simulink model "cpg_optimized"  (R2016a)
settings: Solver=FixedStepAuto  StartTime=0.0  StopTime=inf  FixedStep=0.04  RelTol=1e-3
values from neighbouring files (symbols this model uses):
  A_f = 0.1    [setup.m]
  ICNotPresent = 1    [setup.m]
  joints_in_use = [j_i_m('l_leg_hpx') j_i_m('l_leg_hpy') j_i_m('l_leg_kny') j_i_m('l_leg_aky') j_i_m('l_leg_akx') j_i_m('l_arm_shx') j_i_m('r_leg_hpx') j_i_m('r_leg_hpy') j_i_m('r_leg_kny') j_i_m('r_leg_aky') j_i_m('r_leg_akx') j_i_m('r_arm_shx')]    [setup.m]
  sigma_f = 2.2    [setup.m]
  sigma_s = 1    [setup.m]
  t_m = 0.1    [setup.m]
  t_s = 2    [setup.m]
undefined symbols (not defined in the file or in its folder): DiscIntNeverNeededParam, get, Position, SendJointCommand, SetThisJoint
libraries: fuzblock x72, dspsnks4 x4, simulink x2, robotlib x2, dspsrcs4 x1, dspindex x1, sldrtlib x1
(part 1 of 2)
settings Model: SimulationMode=accelerator  Creator=batyr  LastModifiedBy=batyr
settings SolverCC: EnableConcurrentExecution=on
settings DataIOCC: FinalStateName=CPGSimFinalState  LimitDataPoints=on  SaveCompleteFinalSimState=on  ReturnWorkspaceOutputs=on
settings OptimizationCC: BlockReduction=off  OptimizeBlockIOStorage=off  BufferReuse=off  GlobalBufferReuse=off  ExpressionFolding=off  LocalBlockOutputs=off  EfficientMapNaN2IntZero=off  OptimizeModelRefInitCode=on  MaxStackSize=64
settings DebuggingCC: ReadBeforeWriteMsg=DisableAll  WriteAfterWriteMsg=DisableAll  WriteAfterReadMsg=DisableAll  MultiTaskDSMMsg=none  AllowSymbolicDim=off
settings HardwareCC: ProdBitPerLong=64  ProdLargestAtomicFloat=None  ProdHWDeviceType=Intel->x86-64  TargetBitPerPointer=64  TargetLongLongMode=on  TargetIntDivRoundTo=Zero  TargetEndianess=LittleEndian  TargetWordSize=64  TargetHWDeviceType=MATLAB Host  ProdEqTarget=off
settings ModelReferenceCC: UpdateModelReferenceTargets=IfOutOfDate  PropagateSignalLabelsOutOfModel=off
settings SFSimCC: SFSimEcho=off
settings RTWCC: TargetLang=C++
settings CodeAppCC: MaxIdLength=128
settings GRTTargetCC: GeneratePreprocessorConditionals=Use local settings  CombineOutputUpdateFcns=off  GRTInterface=on

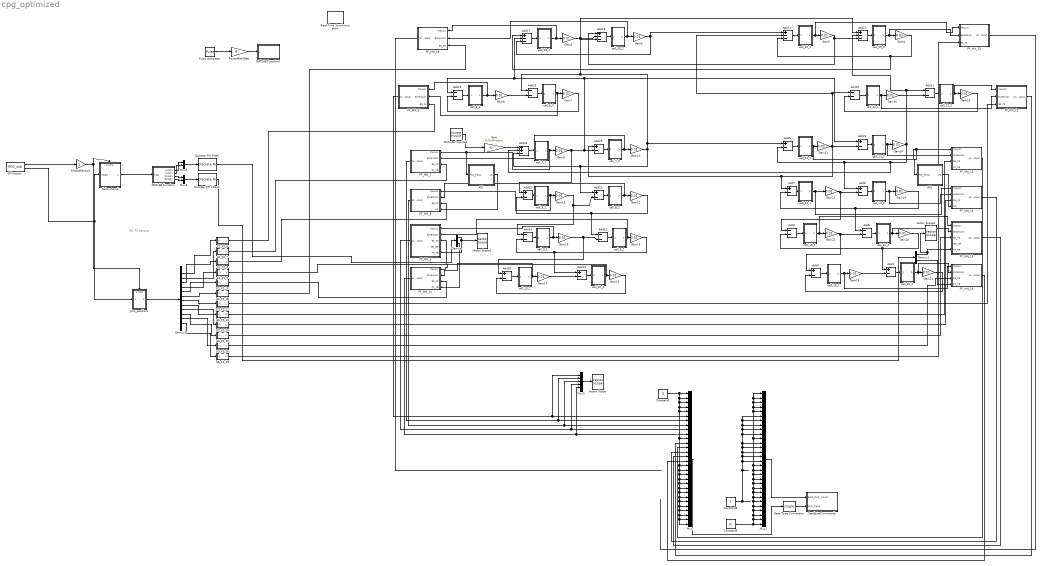
== system cpg_optimized ==
  note: ES, FS sensors
  AS1 : Subsystem
  AS2 : Subsystem
  Add{3,6,10..11,14..16,21} (8 alike) : Sum  Inputs=--
  Add{12..13,17..18} (4 alike) : Sum  Inputs=+--
  Add{4..5,7..9,19..20,22..23,25..26} (11 alike) : Sum  Inputs=+-
  Add24 : Sum  Inputs=++-
  Constant1 : Constant  Value=0  OutDataTypeStr=double
  Constant5 : Constant  Value=0  OutDataTypeStr=boolean
  Constant6 : Constant  OutDataTypeStr=boolean
  Data Type Conversion : DataTypeConversion  OutDataTypeStr=single
  Demux : Demux  Outputs=2
  Demux1 : Demux  Outputs=2
  Demux2 : Demux  Outputs=12
  Discrete Impulse2 : dspsrcs4/Discrete  Impulse  Delay=1  SampleTime=-1  FrameSample=1  OutputFrames=off  dataType=double  isSigned=on  wordLen=16  udDataType=sfix(16)  fracBitsMode=Best precision  numFracBits=15  OutDataTypeStr=double  LastOutDataTypeStr=double
  Discrete FIR Filter : DiscreteFir
  Discrete FIR Filter1 : DiscreteFir
  ES_FS_10 : Subsystem
  ES_FS_12 : Subsystem
  ES_FS_13 : Subsystem
  ES_FS_14 : Subsystem
  ES_FS_15 : Subsystem
  ES_FS_16 : Subsystem
  ES_FS_18 : Subsystem
  ES_FS_25 : Subsystem
  ES_FS_6 : Subsystem
  ES_FS_7 : Subsystem
  ES_FS_8 : Subsystem
  ES_FS_9 : Subsystem
  EnableSensors : Gain
  Gain : Gain  Gain=ICNotPresent
  Gain{3..26} (24 alike) : Gain  Gain=0.01
  Joint_positions : Subsystem
  MATLAB Function : MATLAB Function  TreatAsAtomicUnit=on
  MATLAB Function1 : MATLAB Function  TreatAsAtomicUnit=on
  Mux : Mux  Inputs=30
  Mux2 : Mux  Inputs=30
  Mux3 : Mux  Inputs=2
  Mux4 : Mux  Inputs=2
  Mux5 : Mux  Inputs=5
  PF_MN_10 : Subsystem
  PF_MN_12 : Subsystem
  PF_MN_13 : Subsystem
  PF_MN_14 : Subsystem
  PF_MN_15 : Subsystem
  PF_MN_16 : Subsystem
  PF_MN_18 : Subsystem
  PF_MN_25 : Subsystem
  PF_MN_6 : Subsystem
  PF_MN_7 : Subsystem
  PF_MN_8 : Subsystem
  PF_MN_9 : Subsystem
  PauseAfterStep : Gain  Gain=0
  Pulse Generator : DiscretePulseGenerator  PhaseDelay=1  SampleTime=-1
  Real-Time Synchronization : sldrtlib/Real-Time Synchronization  SampleTime=-1  MaxMissedTicks=100000  ShowMissedTicks=off  YieldWhenWaiting=off
  S-Function : S-Function  FunctionName=ROS_sub  SFunctionDeploymentMode=off  EnableBusSupport=off
  SendJointCommands : Subsystem
  Subsystem4 : Subsystem
  Vector Scope : dspsnks4/Vector Scope  ScopeProperties=on  Domain=Time  HorizSpan=1  DisplayProperties=off  AxisGrid=on  Memory=off  FrameNumber=on  AxisLegend=off  AxisZoom=off  OpenScopeAtSimStart=on  OpenScopeImmediately=off  FigPos=get(0,'defaultfigureposition')  AxisProperties=off  XUnits=Hertz  XRange=[0...Fs/2]  InheritXIncr=on  XIncr=1  XLabel=Time  XLimit=Auto  XMin=0  XMax=1  XStart=0  YUnits=dB  YLabel=Amplitude  LineProperties=off  XAxisParamsVer=6.9
      settings: YMin=-10  YMax=10
  Vector Scope1 : dspsnks4/Vector Scope  ScopeProperties=on  Domain=Time  HorizSpan=1  DisplayProperties=off  AxisGrid=on  Memory=off  FrameNumber=on  AxisLegend=off  AxisZoom=off  OpenScopeAtSimStart=on  OpenScopeImmediately=off  FigPos=get(0,'defaultfigureposition')  AxisProperties=off  XUnits=Hertz  XRange=[0...Fs/2]  InheritXIncr=on  XIncr=1  XLabel=Time  XLimit=Auto  XMin=0  XMax=1  XStart=0  YUnits=dB  YLabel=Amplitude  LineProperties=off  XAxisParamsVer=6.9
      settings: YMin=-10  YMax=10
  Vector Scope2 : dspsnks4/Vector Scope  ScopeProperties=on  Domain=Time  HorizSpan=1  DisplayProperties=off  AxisGrid=on  Memory=off  FrameNumber=on  AxisLegend=off  AxisZoom=off  OpenScopeAtSimStart=on  OpenScopeImmediately=off  FigPos=get(0,'defaultfigureposition')  AxisProperties=off  XUnits=Hertz  XRange=[0...Fs/2]  InheritXIncr=on  XIncr=1  XLabel=Time  XLimit=Auto  XMin=0  XMax=1  XStart=0  YUnits=dB  YLabel=Amplitude  LineProperties=off  XAxisParamsVer=6.9
      settings: YMin=-10  YMax=10
  cell_10_1 : Subsystem
  cell_10_2 : Subsystem
  cell_12_1 : Subsystem
  cell_12_2 : Subsystem
  cell_13_1 : Subsystem
  cell_13_2 : Subsystem
  cell_14_1 : Subsystem
  cell_14_2 : Subsystem
  cell_15_1 : Subsystem
  cell_15_2 : Subsystem
  cell_16_1 : Subsystem
  cell_16_2 : Subsystem
  cell_18_1 : Subsystem
  cell_18_2 : Subsystem
  cell_25_1 : Subsystem
  cell_25_2 : Subsystem
  cell_6_1 : Subsystem
  cell_6_2 : Subsystem
  cell_7_1 : Subsystem
  cell_7_2 : Subsystem
  cell_8_1 : Subsystem
  cell_8_2 : Subsystem
  cell_9_1 : Subsystem
  cell_9_2 : Subsystem
  wires:
  Add3/1 -> cell_15_1/1(In1)
  cell_15_2/1(Out1) -> PF_MN_15/2(Extension), Gain20/1
  cell_15_1/1(Out1) -> PF_MN_15/1(Flexion), Gain22/1
  cell_16_1/1(Out1) -> PF_MN_16/1(Flexion), Gain18/1
  cell_16_2/1(Out1) -> PF_MN_16/2(Extension), Gain21/1
  Add4/1 -> cell_16_2/1(In1)
  Add5/1 -> cell_16_1/1(In1)
  Add6/1 -> cell_15_2/1(In1)
  Add7/1 -> cell_14_1/1(In1)
  cell_14_2/1(Out1) -> PF_MN_14/2(Extension), Gain19/1
  cell_14_1/1(Out1) -> PF_MN_14/1(Flexion), Gain23/1
  Add8/1 -> cell_14_2/1(In1)
  Add9/1 -> cell_13_1/1(In1)
  Add26/1 -> cell_13_2/1(In1)
  cell_7_1/1(Out1) -> AS1/1(Hip_flexor), PF_MN_7/1(Flexion), Gain9/1
  cell_7_2/1(Out1) -> PF_MN_7/2(Extension), Gain10/1
  cell_12_2/1(Out1) -> PF_MN_12/1(Flexion), Gain25/1
  cell_12_1/1(Out1) -> PF_MN_12/2(Extension), Gain26/1
  Add10/1 -> cell_12_1/1(In1)
  Add11/1 -> cell_12_2/1(In1)
  Add12/1 -> cell_25_1/1(In1)
  Add13/1 -> cell_25_2/1(In1)
  Add14/1 -> cell_9_1/1(In1)
  cell_9_2/1(Out1) -> Gain13/1, PF_MN_9/2(Extension)
  cell_9_1/1(Out1) -> PF_MN_9/1(Flexion), Gain16/1
  cell_10_1/1(Out1) -> PF_MN_10/2(Extension), Gain17/1
  cell_10_2/1(Out1) -> PF_MN_10/1(Flexion), Gain14/1
  Add19/1 -> cell_10_2/1(In1)
  Add20/1 -> cell_10_1/1(In1)
  Add21/1 -> cell_9_2/1(In1)
  Add22/1 -> cell_8_1/1(In1)
  cell_8_2/1(Out1) -> PF_MN_8/2(Extension), Gain12/1
  cell_8_1/1(Out1) -> PF_MN_8/1(Flexion), Gain15/1
  Add23/1 -> cell_8_2/1(In1)
  Add24/1 -> cell_7_1/1(In1)
  Add25/1 -> cell_7_2/1(In1)
  cell_13_1/1(Out1) -> AS2/1(Hip_flexor), PF_MN_13/1(Flexion), Gain11/1
  cell_13_2/1(Out1) -> PF_MN_13/2(Extension), Gain24/1
  cell_6_2/1(Out1) -> PF_MN_6/2(Extension), Gain7/1
  cell_6_1/1(Out1) -> PF_MN_6/1(Flexion), Gain8/1
  Add15/1 -> cell_6_1/1(In1)
  Add16/1 -> cell_6_2/1(In1)
  Add17/1 -> cell_18_1/1(In1)
  Discrete Impulse2/1 -> Gain/1
  Add18/1 -> cell_18_2/1(In1)
  cell_18_1/1(Out1) -> PF_MN_18/1(Flexion), Gain3/1
  cell_18_2/1(Out1) -> PF_MN_18/2(Extension), Gain6/1
  cell_25_1/1(Out1) -> PF_MN_25/1(Flexion), Gain5/1
  cell_25_2/1(Out1) -> PF_MN_25/2(Extension), Gain4/1
  Gain3/1 -> Add13/1, Add18/2
  Gain4/1 -> Add17/1, Add12/3
  Gain5/1 -> Add18/1, Add13/3
  Gain6/1 -> Add12/1, Add17/3
  Gain7/1 -> Add15/2
  Gain8/1 -> Add16/2
  Gain9/1 -> Add15/1, Add17/2, Add26/1, Add25/2, Add22/1
  Gain10/1 -> Add18/3, Add16/1, Add9/1, Add24/3, Add23/1
  Gain11/1 -> Add12/2, Add10/1, Add7/1, Add25/1, Add26/2
  Gain12/1 -> Add22/2, Add21/1
  Gain13/1 -> Add14/2, Add19/1
  Gain14/1 -> Add20/2
  Gain15/1 -> Add14/1, Add23/2
  Gain16/1 -> Add20/1, Add21/2
  Gain17/1 -> Add19/2
  Gain18/1 -> Add4/2
  Gain19/1 -> Add7/2, Add6/1
  Gain20/1 -> Add3/2, Add4/1
  Gain21/1 -> Add5/2
  Gain22/1 -> Add6/2, Add5/1
  Gain23/1 -> Add8/2, Add3/1
  Gain24/1 -> Add24/2, Add8/1, Add9/2, Add13/2, Add11/1
  Gain25/1 -> Add10/2
  Gain26/1 -> Add11/2
  S-Function/2 -> Subsystem4/1(MsgIn), Joint_positions/1(Msg)
  Mux/1 -> Data Type Conversion/1
  Joint_positions/1(Out2) -> Demux2/1
  Demux2/1 -> ES_FS_6/1(In)
  Demux2/2 -> ES_FS_7/1(In)
  Demux2/4 -> ES_FS_9/1(In)
  Demux2/5 -> ES_FS_10/1(In)
  Demux2/6 -> ES_FS_18/1(In)
  Demux2/7 -> ES_FS_12/1(In)
  Demux2/8 -> ES_FS_13/1(In)
  Demux2/9 -> ES_FS_14/1(In)
  Demux2/10 -> ES_FS_15/1(In)
  Demux2/11 -> ES_FS_16/1(In)
  Demux2/12 -> ES_FS_25/1(In)
  Demux2/3 -> ES_FS_8/1(In)
  ES_FS_6/1(Out) -> PF_MN_6/3(ES_FS)
  ES_FS_7/1(Out) -> PF_MN_7/3(ES_FS)
  ES_FS_8/1(Out) -> PF_MN_8/3(ES_FS)
  ES_FS_9/1(Out) -> PF_MN_9/3(ES_FS)
  ES_FS_10/1(Out) -> PF_MN_10/3(ES_FS)
  ES_FS_18/1(Out) -> PF_MN_18/3(ES_FS)
  ES_FS_12/1(Out) -> PF_MN_12/3(ES_FS)
  ES_FS_13/1(Out) -> PF_MN_13/3(ES_FS)
  ES_FS_14/1(Out) -> PF_MN_14/3(ES_FS)
  ES_FS_15/1(Out) -> PF_MN_15/3(ES_FS)
  ES_FS_16/1(Out) -> PF_MN_16/3(ES_FS)
  ES_FS_25/1(Out) -> PF_MN_25/3(ES_FS)
  Mux2/1 -> SendJointCommands/1(Send_Joint_Value?)
  AS2/1(AS) -> PF_MN_14/4(AS)
  PF_MN_25/1(Joint_Output) -> ?
  PF_MN_12/1(Joint_Output) -> Mux/12
  PF_MN_13/1(Joint_Output) -> Mux/13
  PF_MN_14/1(Joint_Output) -> Mux/14
  PF_MN_15/1(Joint_Output) -> Mux/15
  PF_MN_16/1(Joint_Output) -> Mux/16
  PF_MN_6/1(Joint_Output) -> Mux5/1, Mux/6
  PF_MN_7/1(Joint_Output) -> Mux5/2, Mux/7
  PF_MN_8/1(Joint_Output) -> Mux5/3, Mux/8
  PF_MN_9/1(Joint_Output) -> Mux5/4, Mux/9
  PF_MN_10/1(Joint_Output) -> Mux5/5, Mux/10
  PF_MN_18/1(Joint_Output) -> ?
  Data Type Conversion/1 -> SendJointCommands/2(Joint_Value)
  Constant6/1 -> Mux2/16, Mux2/15, Mux2/14, Mux2/13, Mux2/12, Mux2/10, Mux2/9, Mux2/8, Mux2/6, Mux2/7
  Mux5/1 -> Vector Scope/1
  AS1/1(AS) -> PF_MN_8/4(AS)
  Constant5/1 -> Mux2/25, Mux2/18, Mux2/1, Mux2/2, Mux2/3, Mux2/4, Mux2/5, Mux2/11, Mux2/17, Mux2/19, Mux2/20, Mux2/21, Mux2/22, Mux2/23, Mux2/24, Mux2/26, Mux2/27, Mux2/28, Mux2/29, Mux2/30
  S-Function/1 -> EnableSensors/1
  Gain/1 -> Add24/1
  EnableSensors/1 -> Joint_positions/Enable, Subsystem4/Enable
  Mux4/1 -> Discrete FIR Filter/1
  Mux3/1 -> Discrete FIR Filter1/1
  Demux1/2 -> PF_MN_16/4(FF_FB)
  Demux1/1 -> Vector Scope2/1, PF_MN_15/5(FF_FB)
  MATLAB Function/3(RFootX) -> Mux3/1
  MATLAB Function/4(RFootY) -> Mux3/2
  MATLAB Function/1(LFootX) -> Mux4/1
  MATLAB Function/2(LFootY) -> Mux4/2
  Demux/1 -> Vector Scope1/1, PF_MN_9/5(FF_FB)
  Demux/2 -> PF_MN_10/4(FF_FB)
  Constant1/1 -> Mux/3, Mux/5, Mux/11, Mux/17, Mux/18, Mux/19, Mux/20, Mux/21, Mux/22, Mux/23, Mux/25, Mux/26, Mux/27, Mux/30, Mux/29, Mux/28, Mux/24, Mux/4, Mux/2, Mux/1
  Pulse Generator/1 -> PauseAfterStep/1
  PauseAfterStep/1 -> MATLAB Function1/1(u)
  Subsystem4/1(MsgOut) -> MATLAB Function/1(msg)
  Discrete FIR Filter/1 -> Demux/1
  Discrete FIR Filter1/1 -> Demux1/1

== system cpg_optimized/AS1 ==
  Hip_flexor : Inport
  Constant1 : Constant  Value=0
  Constant2 : Constant  Value=0.1
  Detect Decrease : simulink/Logic and Bit Operations/Detect Decrease  vinit=1  InputProcessing=Inherited  OutDataTypeStr=boolean
  Display2 : Display
  Display4 : Display
  If : If  IfExpression=u1
  If Action Subsystem1 : Subsystem  TreatAsAtomicUnit=on
  If Action Subsystem3 : Subsystem  TreatAsAtomicUnit=on
  Merge1 : Merge
  AS : Outport
  wires:
  If/2 -> If Action Subsystem1/Action
  Constant1/1 -> If Action Subsystem1/1(In1)
  If Action Subsystem1/1(Out1) -> Merge1/2
  Merge1/1 -> Display2/1, AS/1
  Hip_flexor/1 -> Detect Decrease/1, Display4/1
  Detect Decrease/1 -> If/1
  Constant2/1 -> If Action Subsystem3/1(In1)
  If/1 -> If Action Subsystem3/Action
  If Action Subsystem3/1(Out1) -> Merge1/1

== system cpg_optimized/AS2 ==
  Hip_flexor : Inport
  Constant1 : Constant  Value=0
  Constant2 : Constant  Value=0.1
  Detect Decrease : simulink/Logic and Bit Operations/Detect Decrease  vinit=0.0  InputProcessing=Inherited  OutDataTypeStr=boolean
  Display2 : Display
  Display4 : Display
  If : If  IfExpression=u1
  If Action Subsystem1 : Subsystem  TreatAsAtomicUnit=on
  If Action Subsystem3 : Subsystem  TreatAsAtomicUnit=on
  Merge1 : Merge
  AS : Outport
  wires:
  If/2 -> If Action Subsystem1/Action
  Constant1/1 -> If Action Subsystem1/1(In1)
  If Action Subsystem1/1(Out1) -> Merge1/2
  Merge1/1 -> Display2/1, AS/1
  Hip_flexor/1 -> Detect Decrease/1, Display4/1
  Detect Decrease/1 -> If/1
  Constant2/1 -> If Action Subsystem3/1(In1)
  If/1 -> If Action Subsystem3/Action
  If Action Subsystem3/1(Out1) -> Merge1/1

== system cpg_optimized/ES_FS_10 ==
  In : Inport
  ES : fuzblock/Membership  Functions/Sigmoidal MF  a=6.9767  c=-0.075465
  FS : fuzblock/Membership  Functions/Sigmoidal MF  a=-6.9767  c=-0.075465
  Mux : Mux  Inputs=2
  Out : Outport
  wires:
  FS/1 -> Mux/2
  In/1 -> ES/1, FS/1
  ES/1 -> Mux/1
  Mux/1 -> Out/1

== system cpg_optimized/ES_FS_12 ==
  In : Inport
  ES : fuzblock/Membership  Functions/Sigmoidal MF  a=5.7692  c=-0.075739
  FS : fuzblock/Membership  Functions/Sigmoidal MF  a=-5.7692  c=-0.075739
  Mux : Mux  Inputs=2
  Out : Outport
  wires:
  FS/1 -> Mux/2
  In/1 -> ES/1, FS/1
  ES/1 -> Mux/1
  Mux/1 -> Out/1

== system cpg_optimized/ES_FS_13 ==
  In : Inport
  ES : fuzblock/Membership  Functions/Sigmoidal MF  a=2.765  c=-0.2
  FS : fuzblock/Membership  Functions/Sigmoidal MF  a=-2.765  c=-0.2
  Mux : Mux  Inputs=2
  Out : Outport
  wires:
  FS/1 -> Mux/2
  In/1 -> ES/1, FS/1
  ES/1 -> Mux/1
  Mux/1 -> Out/1

== system cpg_optimized/ES_FS_14 ==
  In : Inport
  ES : fuzblock/Membership  Functions/Sigmoidal MF  a=-2.5532  c=0.45
  FS : fuzblock/Membership  Functions/Sigmoidal MF  a=2.5532  c=0.45
  Mux : Mux  Inputs=2
  Out : Outport
  wires:
  FS/1 -> Mux/2
  In/1 -> ES/1, FS/1
  ES/1 -> Mux/1
  Mux/1 -> Out/1

== system cpg_optimized/ES_FS_15 ==
  In : Inport
  ES : fuzblock/Membership  Functions/Sigmoidal MF  a=4.3478  c=-0.1
  FS : fuzblock/Membership  Functions/Sigmoidal MF  a=-4.3478  c=-0.1
  Mux : Mux  Inputs=2
  Out : Outport
  wires:
  FS/1 -> Mux/2
  In/1 -> ES/1, FS/1
  ES/1 -> Mux/1
  Mux/1 -> Out/1

== system cpg_optimized/ES_FS_16 ==
  In : Inport
  ES : fuzblock/Membership  Functions/Sigmoidal MF  a=6.9767  c=0.076658
  FS : fuzblock/Membership  Functions/Sigmoidal MF  a=-6.9767  c=0.076658
  Mux : Mux  Inputs=2
  Out : Outport
  wires:
  FS/1 -> Mux/2
  In/1 -> ES/1, FS/1
  ES/1 -> Mux/1
  Mux/1 -> Out/1

== system cpg_optimized/ES_FS_18 ==
  In : Inport
  ES : fuzblock/Membership  Functions/Sigmoidal MF  a=1.9108  c=-1.3087
  FS : fuzblock/Membership  Functions/Sigmoidal MF  a=-1.9108  c=-1.3087
  Mux : Mux  Inputs=2
  Out : Outport
  wires:
  FS/1 -> Mux/2
  In/1 -> ES/1, FS/1
  ES/1 -> Mux/1
  Mux/1 -> Out/1

== system cpg_optimized/ES_FS_25 ==
  In : Inport
  ES : fuzblock/Membership  Functions/Sigmoidal MF  a=1.9108  c=1.3088
  FS : fuzblock/Membership  Functions/Sigmoidal MF  a=-1.9108  c=1.3088
  Mux : Mux  Inputs=2
  Out : Outport
  wires:
  FS/1 -> Mux/2
  In/1 -> ES/1, FS/1
  ES/1 -> Mux/1
  Mux/1 -> Out/1

== system cpg_optimized/ES_FS_6 ==
  In : Inport
  Display : Display
  ES : fuzblock/Membership  Functions/Sigmoidal MF  a=5.7692  c=0.075814
  FS : fuzblock/Membership  Functions/Sigmoidal MF  a=-5.7692  c=0.075814
  Mux : Mux  Inputs=2
  Out : Outport
  wires:
  FS/1 -> Mux/2
  In/1 -> ES/1, FS/1
  ES/1 -> Display/1, Mux/1
  Mux/1 -> Out/1

== system cpg_optimized/ES_FS_7 ==
  In : Inport
  ES : fuzblock/Membership  Functions/Sigmoidal MF  a=2.765  c=-0.2
  FS : fuzblock/Membership  Functions/Sigmoidal MF  a=-2.765  c=-0.2
  Mux : Mux  Inputs=2
  Out : Outport
  wires:
  FS/1 -> Mux/2
  In/1 -> ES/1, FS/1
  ES/1 -> Mux/1
  Mux/1 -> Out/1

== system cpg_optimized/ES_FS_8 ==
  In : Inport
  ES : fuzblock/Membership  Functions/Sigmoidal MF  a=-2.5532  c=0.45
  FS : fuzblock/Membership  Functions/Sigmoidal MF  a=2.5532  c=0.45
  Mux : Mux  Inputs=2
  Out : Outport
  wires:
  FS/1 -> Mux/2
  In/1 -> ES/1, FS/1
  ES/1 -> Mux/1
  Mux/1 -> Out/1

== system cpg_optimized/ES_FS_9 ==
  In : Inport
  ES : fuzblock/Membership  Functions/Sigmoidal MF  a=4.3478  c=-0.1
  FS : fuzblock/Membership  Functions/Sigmoidal MF  a=-4.3478  c=-0.1
  Mux : Mux  Inputs=2
  Out : Outport
  wires:
  FS/1 -> Mux/2
  In/1 -> ES/1, FS/1
  ES/1 -> Mux/1
  Mux/1 -> Out/1

== system cpg_optimized/Joint_positions ==
  Msg : Inport
  Enable : EnablePort
  Bus Selector : BusSelector  OutputSignals=Joints
  Constant7 : Constant  Value=joints_in_use
  Variable Selector2 : dspindex/Variable Selector  NumInputs=1  rowsOrCols=Rows  IdxMode=Variable  Elements=[1 3]  ZerOneIdxMode=One-based  errmode=Clip Index  FillMode=on  FillValues=0
  Vector Scope : dspsnks4/Vector Scope  ScopeProperties=on  Domain=Time  HorizSpan=1  DisplayProperties=off  AxisGrid=on  Memory=off  FrameNumber=on  AxisLegend=off  AxisZoom=off  OpenScopeAtSimStart=on  OpenScopeImmediately=off  FigPos=get(0,'defaultfigureposition')  AxisProperties=off  XUnits=Hertz  XRange=[0...Fs/2]  InheritXIncr=on  XIncr=1  XLabel=Time  XLimit=Auto  XMin=0  XMax=1  XStart=0  YUnits=dB  YLabel=Amplitude  LineProperties=off  XAxisParamsVer=6.9
      settings: YMin=-10  YMax=10
  Out2 : Outport
  wires:
  Constant7/1 -> Variable Selector2/2
  Variable Selector2/1 -> Out2/1
  Msg/1 -> Bus Selector/1
  Bus Selector/1 -> Vector Scope/1, Variable Selector2/1  "<Joints>"

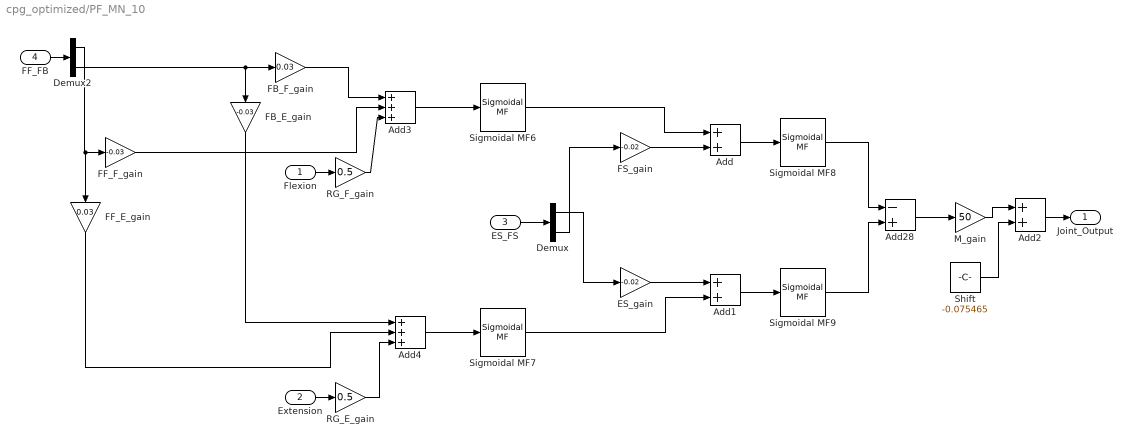
== system cpg_optimized/PF_MN_10 ==
  Flexion : Inport
  Extension : Inport  Port=2
  ES_FS : Inport  Port=3
  FF_FB : Inport  Port=4
  Add : Sum
  Add1 : Sum
  Add2 : Sum
  Add28 : Sum  Inputs=-+
  Add3 : Sum  Inputs=+++
  Add4 : Sum  Inputs=+++
  Demux : Demux  Outputs=2
  Demux2 : Demux  Outputs=2
  ES_gain : Gain  Gain=-0.02
  FB_E_gain : Gain  Gain=-0.03
  FB_F_gain : Gain  Gain=0.03
  FF_E_gain : Gain  Gain=0.03
  FF_F_gain : Gain  Gain=-0.03
  FS_gain : Gain  Gain=-0.02
  M_gain : Gain  Gain=50
  RG_E_gain : Gain  Gain=0.5
  RG_F_gain : Gain  Gain=0.5
  Shift : Constant  Value=-0.075465
  Sigmoidal MF{6..9} (4 alike) : fuzblock/Membership  Functions/Sigmoidal MF  a=1  c=0
  Joint_Output : Outport
  wires:
  Extension/1 -> RG_E_gain/1
  Sigmoidal MF6/1 -> Add/1
  Sigmoidal MF7/1 -> Add1/2
  Flexion/1 -> RG_F_gain/1
  ES_FS/1 -> Demux/1
  Sigmoidal MF9/1 -> Add28/2
  Sigmoidal MF8/1 -> Add28/1
  Add28/1 -> M_gain/1
  Add1/1 -> Sigmoidal MF9/1
  Add/1 -> Sigmoidal MF8/1
  FS_gain/1 -> Add/2
  ES_gain/1 -> Add1/1
  Demux/2 -> FS_gain/1
  Demux/1 -> ES_gain/1
  M_gain/1 -> Add2/1
  Shift/1 -> Add2/2
  Add2/1 -> Joint_Output/1
  FF_FB/1 -> Demux2/1
  Demux2/1 -> FF_E_gain/1, FF_F_gain/1
  Demux2/2 -> FB_E_gain/1, FB_F_gain/1
  FB_F_gain/1 -> Add3/1
  FB_E_gain/1 -> Add4/1
  FF_F_gain/1 -> Add3/2
  FF_E_gain/1 -> Add4/2
  Add3/1 -> Sigmoidal MF6/1
  Add4/1 -> Sigmoidal MF7/1
  RG_F_gain/1 -> Add3/3
  RG_E_gain/1 -> Add4/3

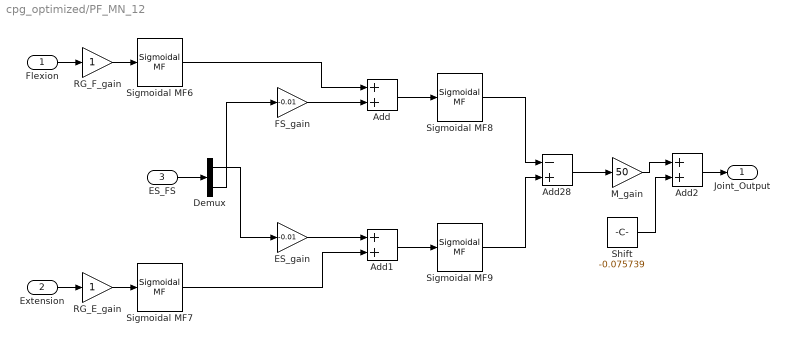
== system cpg_optimized/PF_MN_12 ==
  Flexion : Inport
  Extension : Inport  Port=2
  ES_FS : Inport  Port=3
  Add : Sum
  Add1 : Sum
  Add2 : Sum
  Add28 : Sum  Inputs=-+
  Demux : Demux  Outputs=2
  ES_gain : Gain  Gain=-0.01
  FS_gain : Gain  Gain=-0.01
  M_gain : Gain  Gain=50
  RG_E_gain : Gain
  RG_F_gain : Gain
  Shift : Constant  Value=-0.075739
  Sigmoidal MF{6..9} (4 alike) : fuzblock/Membership  Functions/Sigmoidal MF  a=1  c=0
  Joint_Output : Outport
  wires:
  Extension/1 -> RG_E_gain/1
  Sigmoidal MF6/1 -> Add/1
  Sigmoidal MF7/1 -> Add1/2
  Flexion/1 -> RG_F_gain/1
  ES_FS/1 -> Demux/1
  Sigmoidal MF9/1 -> Add28/2
  Sigmoidal MF8/1 -> Add28/1
  Add28/1 -> M_gain/1
  Add1/1 -> Sigmoidal MF9/1
  Add/1 -> Sigmoidal MF8/1
  FS_gain/1 -> Add/2
  ES_gain/1 -> Add1/1
  Demux/2 -> FS_gain/1
  Demux/1 -> ES_gain/1
  M_gain/1 -> Add2/1
  Shift/1 -> Add2/2
  Add2/1 -> Joint_Output/1
  RG_E_gain/1 -> Sigmoidal MF7/1
  RG_F_gain/1 -> Sigmoidal MF6/1

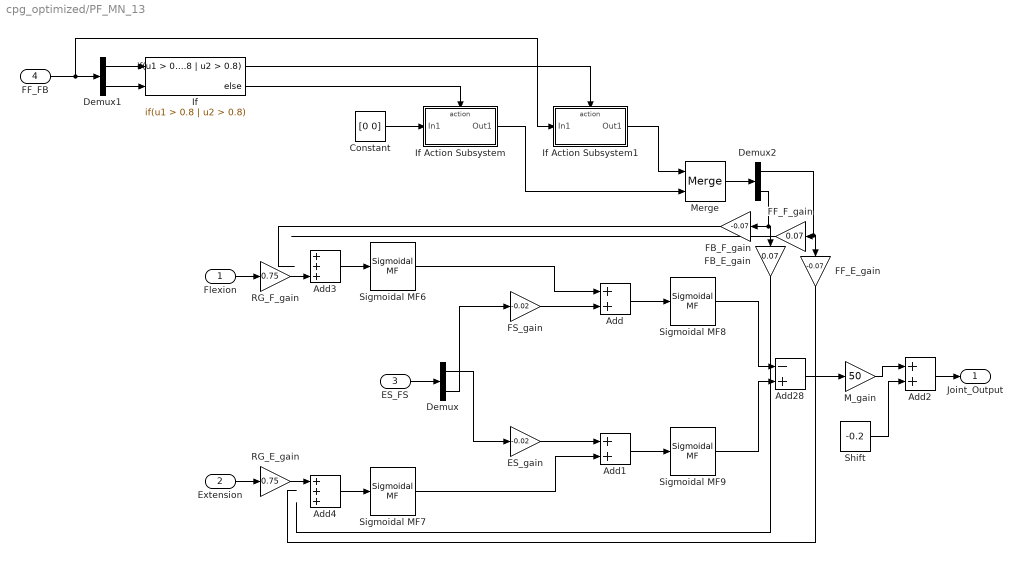
== system cpg_optimized/PF_MN_13 ==
  Flexion : Inport
  Extension : Inport  Port=2
  ES_FS : Inport  Port=3
  FF_FB : Inport  Port=4
  Add : Sum
  Add1 : Sum
  Add2 : Sum
  Add28 : Sum  Inputs=-+
  Add3 : Sum  Inputs=+++
  Add4 : Sum  Inputs=+++
  Constant : Constant  Value=[0 0]
  Demux : Demux  Outputs=2
  Demux1 : Demux  Outputs=2
  Demux2 : Demux  Outputs=2
  ES_gain : Gain  Gain=-0.02
  FB_E_gain : Gain  Gain=0.07
  FB_F_gain : Gain  Gain=-0.07
  FF_E_gain : Gain  Gain=-0.07
  FF_F_gain : Gain  Gain=0.07
  FS_gain : Gain  Gain=-0.02
  If : If  NumInputs=2  IfExpression=u1 > 0.8 | u2 > 0.8
  If Action Subsystem : Subsystem  TreatAsAtomicUnit=on
  If Action Subsystem1 : Subsystem  TreatAsAtomicUnit=on
  M_gain : Gain  Gain=50
  Merge : Merge
  RG_E_gain : Gain  Gain=0.75
  RG_F_gain : Gain  Gain=0.75
  Shift : Constant  Value=-0.2
  Sigmoidal MF{6..9} (4 alike) : fuzblock/Membership  Functions/Sigmoidal MF  a=1  c=0
  Joint_Output : Outport
  wires:
  Extension/1 -> RG_E_gain/1
  Sigmoidal MF6/1 -> Add/1
  Sigmoidal MF7/1 -> Add1/2
  Flexion/1 -> RG_F_gain/1
  ES_FS/1 -> Demux/1
  Sigmoidal MF9/1 -> Add28/2
  Sigmoidal MF8/1 -> Add28/1
  Add28/1 -> M_gain/1
  Add1/1 -> Sigmoidal MF9/1
  Add/1 -> Sigmoidal MF8/1
  FS_gain/1 -> Add/2
  ES_gain/1 -> Add1/1
  Demux/2 -> FS_gain/1
  Demux/1 -> ES_gain/1
  M_gain/1 -> Add2/1
  Shift/1 -> Add2/2
  Add2/1 -> Joint_Output/1
  Add3/1 -> Sigmoidal MF6/1
  Add4/1 -> Sigmoidal MF7/1
  FF_FB/1 -> If Action Subsystem1/1(In1), Demux1/1
  Demux1/1 -> If/1
  Demux1/2 -> If/2
  If/2 -> If Action Subsystem/Action
  If/1 -> If Action Subsystem1/Action
  If Action Subsystem1/1(Out1) -> Merge/1
  If Action Subsystem/1(Out1) -> Merge/2
  Constant/1 -> If Action Subsystem/1(In1)
  Merge/1 -> Demux2/1
  Demux2/2 -> FB_E_gain/1, FB_F_gain/1
  Demux2/1 -> FF_E_gain/1, FF_F_gain/1
  FF_E_gain/1 -> ?
  FF_F_gain/1 -> ?
  FB_E_gain/1 -> ?
  FB_F_gain/1 -> ?
  RG_F_gain/1 -> Add3/3
  RG_E_gain/1 -> Add4/1

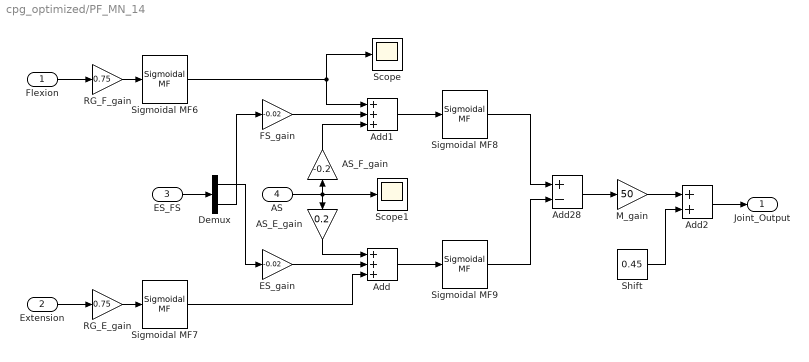
== system cpg_optimized/PF_MN_14 ==
  Flexion : Inport
  Extension : Inport  Port=2
  ES_FS : Inport  Port=3
  AS : Inport  Port=4
  AS_E_gain : Gain  Gain=0.2
  AS_F_gain : Gain  Gain=-0.2
  Add : Sum  Inputs=+++
  Add1 : Sum  Inputs=+++
  Add2 : Sum
  Add28 : Sum  Inputs=+-
  Demux : Demux  Outputs=2
  ES_gain : Gain  Gain=-0.02
  FS_gain : Gain  Gain=-0.02
  M_gain : Gain  Gain=50
  RG_E_gain : Gain  Gain=0.75
  RG_F_gain : Gain  Gain=0.75
  Scope : Scope
  Scope1 : Scope
  Shift : Constant  Value=0.45
  Sigmoidal MF{6..9} (4 alike) : fuzblock/Membership  Functions/Sigmoidal MF  a=1  c=0
  Joint_Output : Outport
  wires:
  Extension/1 -> RG_E_gain/1
  Sigmoidal MF6/1 -> Add1/1, Scope/1
  Flexion/1 -> RG_F_gain/1
  ES_FS/1 -> Demux/1
  Sigmoidal MF9/1 -> Add28/2
  Sigmoidal MF8/1 -> Add28/1
  Add28/1 -> M_gain/1
  M_gain/1 -> Add2/1
  Add/1 -> Sigmoidal MF9/1
  Add1/1 -> Sigmoidal MF8/1
  Demux/2 -> FS_gain/1
  Demux/1 -> ES_gain/1
  AS/1 -> Scope1/1, AS_E_gain/1, AS_F_gain/1
  AS_F_gain/1 -> Add1/3
  AS_E_gain/1 -> Add/1
  Sigmoidal MF7/1 -> Add/3
  Shift/1 -> Add2/2
  Add2/1 -> Joint_Output/1
  FS_gain/1 -> Add1/2
  ES_gain/1 -> Add/2
  RG_F_gain/1 -> Sigmoidal MF6/1
  RG_E_gain/1 -> Sigmoidal MF7/1

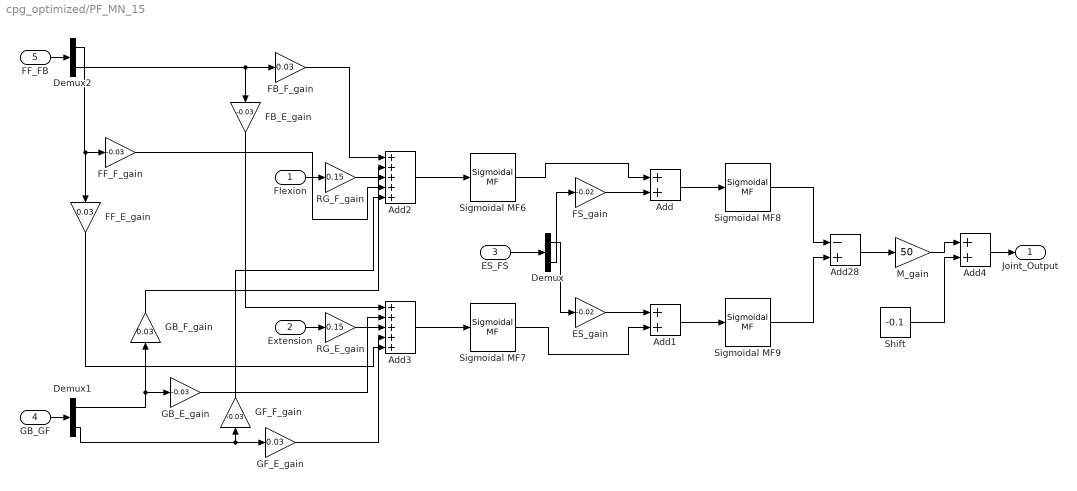
== system cpg_optimized/PF_MN_15 ==
  Flexion : Inport
  Extension : Inport  Port=2
  ES_FS : Inport  Port=3
  GB_GF : Inport  Port=4
  FF_FB : Inport  Port=5
  Add : Sum
  Add1 : Sum
  Add2 : Sum  Inputs=+++++
  Add28 : Sum  Inputs=-+
  Add3 : Sum  Inputs=+++++
  Add4 : Sum
  Demux : Demux  Outputs=2
  Demux1 : Demux  Outputs=2
  Demux2 : Demux  Outputs=2
  ES_gain : Gain  Gain=-0.02
  FB_E_gain : Gain  Gain=-0.03
  FB_F_gain : Gain  Gain=0.03
  FF_E_gain : Gain  Gain=0.03
  FF_F_gain : Gain  Gain=-0.03
  FS_gain : Gain  Gain=-0.02
  GB_E_gain : Gain  Gain=-0.03
  GB_F_gain : Gain  Gain=0.03
  GF_E_gain : Gain  Gain=0.03
  GF_F_gain : Gain  Gain=-0.03
  M_gain : Gain  Gain=50
  RG_E_gain : Gain  Gain=0.15
  RG_F_gain : Gain  Gain=0.15
  Shift : Constant  Value=-0.1
  Sigmoidal MF{6..9} (4 alike) : fuzblock/Membership  Functions/Sigmoidal MF  a=1  c=0
  Joint_Output : Outport
  wires:
  Extension/1 -> RG_E_gain/1
  Flexion/1 -> RG_F_gain/1
  Sigmoidal MF9/1 -> Add28/2
  Sigmoidal MF8/1 -> Add28/1
  Add28/1 -> M_gain/1
  Sigmoidal MF7/1 -> Add1/2
  Add2/1 -> Sigmoidal MF6/1
  Add3/1 -> Sigmoidal MF7/1
  Add1/1 -> Sigmoidal MF9/1
  Add/1 -> Sigmoidal MF8/1
  ES_FS/1 -> Demux/1
  Demux/2 -> FS_gain/1
  Demux/1 -> ES_gain/1
  Sigmoidal MF6/1 -> Add/1
  GB_GF/1 -> Demux1/1
  FF_FB/1 -> Demux2/1
  Demux2/1 -> FF_E_gain/1, FF_F_gain/1
  Demux2/2 -> FB_E_gain/1, FB_F_gain/1
  Demux1/1 -> GB_F_gain/1, GB_E_gain/1
  Demux1/2 -> GF_F_gain/1, GF_E_gain/1
  FS_gain/1 -> Add/2
  ES_gain/1 -> Add1/1
  FB_F_gain/1 -> Add2/1
  FB_E_gain/1 -> Add3/1
  GB_F_gain/1 -> Add2/2
  GB_E_gain/1 -> Add3/2
  GF_E_gain/1 -> Add3/4
  GF_F_gain/1 -> Add2/5
  FF_F_gain/1 -> Add2/4
  FF_E_gain/1 -> Add3/5
  M_gain/1 -> Add4/1
  Shift/1 -> Add4/2
  Add4/1 -> Joint_Output/1
  RG_F_gain/1 -> Add2/3
  RG_E_gain/1 -> Add3/3

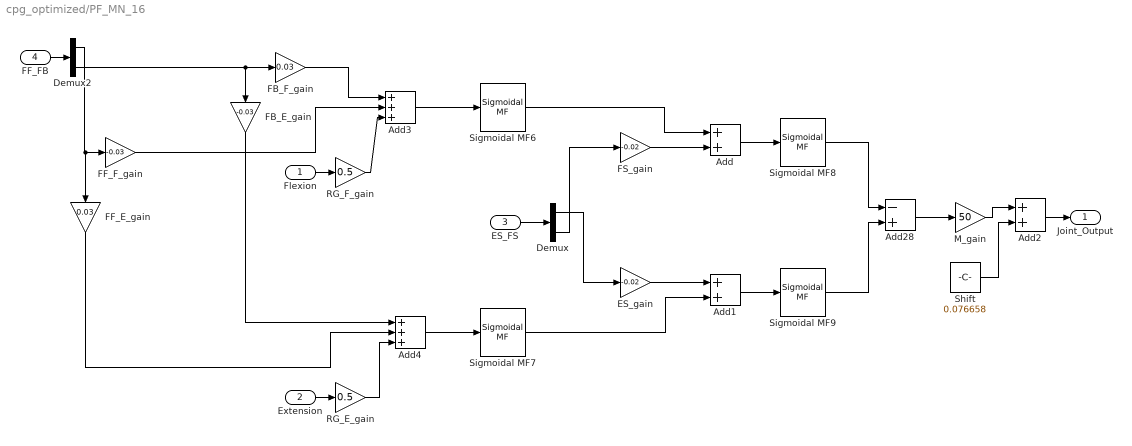
== system cpg_optimized/PF_MN_16 ==
  Flexion : Inport
  Extension : Inport  Port=2
  ES_FS : Inport  Port=3
  FF_FB : Inport  Port=4
  Add : Sum
  Add1 : Sum
  Add2 : Sum
  Add28 : Sum  Inputs=-+
  Add3 : Sum  Inputs=+++
  Add4 : Sum  Inputs=+++
  Demux : Demux  Outputs=2
  Demux2 : Demux  Outputs=2
  ES_gain : Gain  Gain=-0.02
  FB_E_gain : Gain  Gain=-0.03
  FB_F_gain : Gain  Gain=0.03
  FF_E_gain : Gain  Gain=0.03
  FF_F_gain : Gain  Gain=-0.03
  FS_gain : Gain  Gain=-0.02
  M_gain : Gain  Gain=50
  RG_E_gain : Gain  Gain=0.5
  RG_F_gain : Gain  Gain=0.5
  Shift : Constant  Value=0.076658
  Sigmoidal MF{6..9} (4 alike) : fuzblock/Membership  Functions/Sigmoidal MF  a=1  c=0
  Joint_Output : Outport
  wires:
  Extension/1 -> RG_E_gain/1
  Sigmoidal MF6/1 -> Add/1
  Sigmoidal MF7/1 -> Add1/2
  Flexion/1 -> RG_F_gain/1
  ES_FS/1 -> Demux/1
  Sigmoidal MF9/1 -> Add28/2
  Sigmoidal MF8/1 -> Add28/1
  Add28/1 -> M_gain/1
  Add1/1 -> Sigmoidal MF9/1
  Add/1 -> Sigmoidal MF8/1
  FS_gain/1 -> Add/2
  ES_gain/1 -> Add1/1
  Demux/2 -> FS_gain/1
  Demux/1 -> ES_gain/1
  M_gain/1 -> Add2/1
  Shift/1 -> Add2/2
  Add2/1 -> Joint_Output/1
  FF_FB/1 -> Demux2/1
  Demux2/1 -> FF_E_gain/1, FF_F_gain/1
  Demux2/2 -> FB_E_gain/1, FB_F_gain/1
  FB_F_gain/1 -> Add3/1
  FB_E_gain/1 -> Add4/1
  FF_F_gain/1 -> Add3/2
  FF_E_gain/1 -> Add4/2
  Add3/1 -> Sigmoidal MF6/1
  Add4/1 -> Sigmoidal MF7/1
  RG_F_gain/1 -> Add3/3
  RG_E_gain/1 -> Add4/3

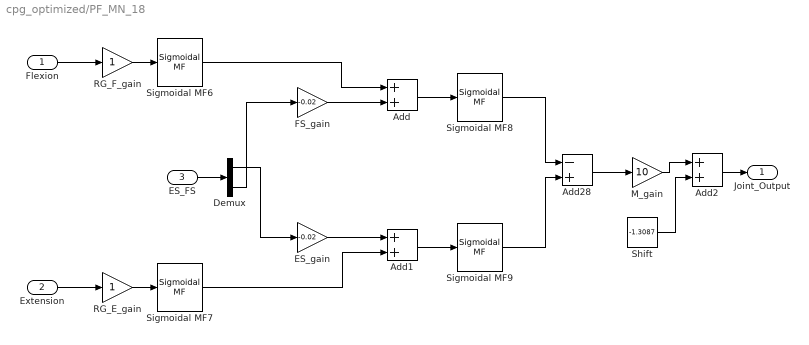
== system cpg_optimized/PF_MN_18 ==
  Flexion : Inport
  Extension : Inport  Port=2
  ES_FS : Inport  Port=3
  Add : Sum
  Add1 : Sum
  Add2 : Sum
  Add28 : Sum  Inputs=-+
  Demux : Demux  Outputs=2
  ES_gain : Gain  Gain=-0.02
  FS_gain : Gain  Gain=-0.02
  M_gain : Gain  Gain=10
  RG_E_gain : Gain
  RG_F_gain : Gain
  Shift : Constant  Value=-1.3087
  Sigmoidal MF{6..9} (4 alike) : fuzblock/Membership  Functions/Sigmoidal MF  a=1  c=0
  Joint_Output : Outport
  wires:
  Extension/1 -> RG_E_gain/1
  Sigmoidal MF6/1 -> Add/1
  Sigmoidal MF7/1 -> Add1/2
  Flexion/1 -> RG_F_gain/1
  ES_FS/1 -> Demux/1
  Sigmoidal MF9/1 -> Add28/2
  Sigmoidal MF8/1 -> Add28/1
  Add28/1 -> M_gain/1
  Add1/1 -> Sigmoidal MF9/1
  Add/1 -> Sigmoidal MF8/1
  FS_gain/1 -> Add/2
  ES_gain/1 -> Add1/1
  Demux/2 -> FS_gain/1
  Demux/1 -> ES_gain/1
  M_gain/1 -> Add2/1
  Shift/1 -> Add2/2
  Add2/1 -> Joint_Output/1
  RG_E_gain/1 -> Sigmoidal MF7/1
  RG_F_gain/1 -> Sigmoidal MF6/1

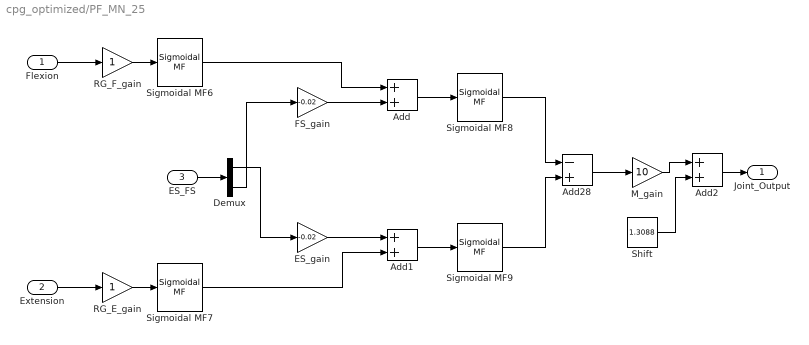
== system cpg_optimized/PF_MN_25 ==
  Flexion : Inport
  Extension : Inport  Port=2
  ES_FS : Inport  Port=3
  Add : Sum
  Add1 : Sum
  Add2 : Sum
  Add28 : Sum  Inputs=-+
  Demux : Demux  Outputs=2
  ES_gain : Gain  Gain=-0.02
  FS_gain : Gain  Gain=-0.02
  M_gain : Gain  Gain=10
  RG_E_gain : Gain
  RG_F_gain : Gain
  Shift : Constant  Value=1.3088
  Sigmoidal MF{6..9} (4 alike) : fuzblock/Membership  Functions/Sigmoidal MF  a=1  c=0
  Joint_Output : Outport
  wires:
  Extension/1 -> RG_E_gain/1
  Sigmoidal MF6/1 -> Add/1
  Sigmoidal MF7/1 -> Add1/2
  Flexion/1 -> RG_F_gain/1
  ES_FS/1 -> Demux/1
  Sigmoidal MF9/1 -> Add28/2
  Sigmoidal MF8/1 -> Add28/1
  Add28/1 -> M_gain/1
  Add1/1 -> Sigmoidal MF9/1
  Add/1 -> Sigmoidal MF8/1
  FS_gain/1 -> Add/2
  ES_gain/1 -> Add1/1
  Demux/2 -> FS_gain/1
  Demux/1 -> ES_gain/1
  M_gain/1 -> Add2/1
  Shift/1 -> Add2/2
  Add2/1 -> Joint_Output/1
  RG_E_gain/1 -> Sigmoidal MF7/1
  RG_F_gain/1 -> Sigmoidal MF6/1

== system cpg_optimized/PF_MN_6 ==
  Flexion : Inport
  Extension : Inport  Port=2
  ES_FS : Inport  Port=3
  Add : Sum
  Add1 : Sum
  Add2 : Sum
  Add28 : Sum  Inputs=-+
  Demux : Demux  Outputs=2
  ES_gain : Gain  Gain=-0.01
  FS_gain : Gain  Gain=-0.01
  M_gain : Gain  Gain=50
  RG_E_gain : Gain
  RG_F_gain : Gain
  Shift : Constant  Value=0.075814
  Sigmoidal MF{6..9} (4 alike) : fuzblock/Membership  Functions/Sigmoidal MF  a=1  c=0
  Joint_Output : Outport
  wires:
  Extension/1 -> RG_E_gain/1
  Sigmoidal MF6/1 -> Add/1
  Sigmoidal MF7/1 -> Add1/2
  Flexion/1 -> RG_F_gain/1
  ES_FS/1 -> Demux/1
  Sigmoidal MF9/1 -> Add28/2
  Sigmoidal MF8/1 -> Add28/1
  Add28/1 -> M_gain/1
  Add1/1 -> Sigmoidal MF9/1
  Add/1 -> Sigmoidal MF8/1
  FS_gain/1 -> Add/2
  ES_gain/1 -> Add1/1
  Demux/2 -> FS_gain/1
  Demux/1 -> ES_gain/1
  M_gain/1 -> Add2/1
  Shift/1 -> Add2/2
  Add2/1 -> Joint_Output/1
  RG_E_gain/1 -> Sigmoidal MF7/1
  RG_F_gain/1 -> Sigmoidal MF6/1

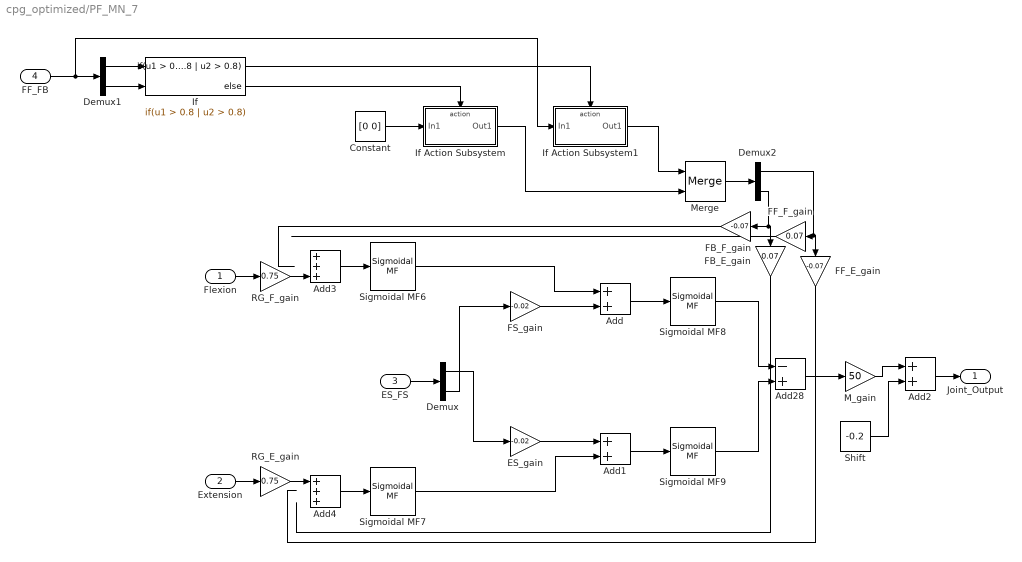
== system cpg_optimized/PF_MN_7 ==
  Flexion : Inport
  Extension : Inport  Port=2
  ES_FS : Inport  Port=3
  FF_FB : Inport  Port=4
  Add : Sum
  Add1 : Sum
  Add2 : Sum
  Add28 : Sum  Inputs=-+
  Add3 : Sum  Inputs=+++
  Add4 : Sum  Inputs=+++
  Constant : Constant  Value=[0 0]
  Demux : Demux  Outputs=2
  Demux1 : Demux  Outputs=2
  Demux2 : Demux  Outputs=2
  ES_gain : Gain  Gain=-0.02
  FB_E_gain : Gain  Gain=0.07
  FB_F_gain : Gain  Gain=-0.07
  FF_E_gain : Gain  Gain=-0.07
  FF_F_gain : Gain  Gain=0.07
  FS_gain : Gain  Gain=-0.02
  If : If  NumInputs=2  IfExpression=u1 > 0.8 | u2 > 0.8
  If Action Subsystem : Subsystem  TreatAsAtomicUnit=on
  If Action Subsystem1 : Subsystem  TreatAsAtomicUnit=on
  M_gain : Gain  Gain=50
  Merge : Merge
  RG_E_gain : Gain  Gain=0.75
  RG_F_gain : Gain  Gain=0.75
  Shift : Constant  Value=-0.2
  Sigmoidal MF{6..9} (4 alike) : fuzblock/Membership  Functions/Sigmoidal MF  a=1  c=0
  Joint_Output : Outport
  wires:
  Extension/1 -> RG_E_gain/1
  Sigmoidal MF6/1 -> Add/1
  Sigmoidal MF7/1 -> Add1/2
  Flexion/1 -> RG_F_gain/1
  ES_FS/1 -> Demux/1
  Sigmoidal MF9/1 -> Add28/2
  Sigmoidal MF8/1 -> Add28/1
  Add28/1 -> M_gain/1
  Add1/1 -> Sigmoidal MF9/1
  Add/1 -> Sigmoidal MF8/1
  FS_gain/1 -> Add/2
  ES_gain/1 -> Add1/1
  Demux/2 -> FS_gain/1
  Demux/1 -> ES_gain/1
  M_gain/1 -> Add2/1
  Shift/1 -> Add2/2
  Add2/1 -> Joint_Output/1
  Add3/1 -> Sigmoidal MF6/1
  Add4/1 -> Sigmoidal MF7/1
  FF_FB/1 -> If Action Subsystem1/1(In1), Demux1/1
  Demux1/1 -> If/1
  Demux1/2 -> If/2
  If/2 -> If Action Subsystem/Action
  If/1 -> If Action Subsystem1/Action
  If Action Subsystem1/1(Out1) -> Merge/1
  If Action Subsystem/1(Out1) -> Merge/2
  Constant/1 -> If Action Subsystem/1(In1)
  Merge/1 -> Demux2/1
  Demux2/2 -> FB_E_gain/1, FB_F_gain/1
  Demux2/1 -> FF_E_gain/1, FF_F_gain/1
  FF_E_gain/1 -> ?
  FF_F_gain/1 -> ?
  FB_E_gain/1 -> ?
  FB_F_gain/1 -> ?
  RG_F_gain/1 -> Add3/3
  RG_E_gain/1 -> Add4/1

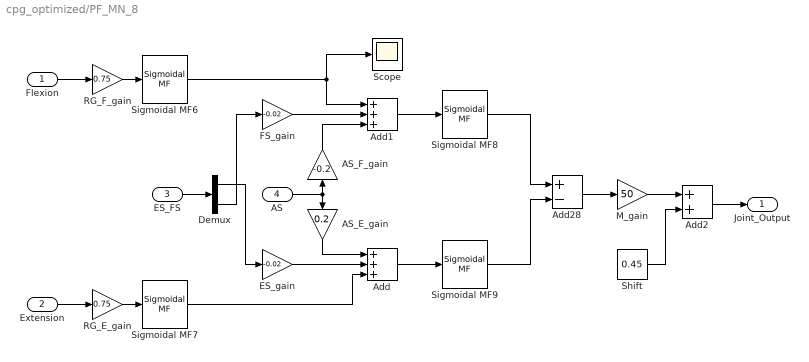
== system cpg_optimized/PF_MN_8 ==
  Flexion : Inport
  Extension : Inport  Port=2
  ES_FS : Inport  Port=3
  AS : Inport  Port=4
  AS_E_gain : Gain  Gain=0.2
  AS_F_gain : Gain  Gain=-0.2
  Add : Sum  Inputs=+++
  Add1 : Sum  Inputs=+++
  Add2 : Sum
  Add28 : Sum  Inputs=+-
  Demux : Demux  Outputs=2
  ES_gain : Gain  Gain=-0.02
  FS_gain : Gain  Gain=-0.02
  M_gain : Gain  Gain=50
  RG_E_gain : Gain  Gain=0.75
  RG_F_gain : Gain  Gain=0.75
  Scope : Scope
  Shift : Constant  Value=0.45
  Sigmoidal MF{6..9} (4 alike) : fuzblock/Membership  Functions/Sigmoidal MF  a=1  c=0
  Joint_Output : Outport
  wires:
  Extension/1 -> RG_E_gain/1
  Sigmoidal MF6/1 -> Add1/1, Scope/1
  Flexion/1 -> RG_F_gain/1
  ES_FS/1 -> Demux/1
  Sigmoidal MF9/1 -> Add28/2
  Sigmoidal MF8/1 -> Add28/1
  Add28/1 -> M_gain/1
  M_gain/1 -> Add2/1
  Add/1 -> Sigmoidal MF9/1
  Add1/1 -> Sigmoidal MF8/1
  Demux/2 -> FS_gain/1
  Demux/1 -> ES_gain/1
  AS/1 -> AS_E_gain/1, AS_F_gain/1
  AS_F_gain/1 -> Add1/3
  AS_E_gain/1 -> Add/1
  Sigmoidal MF7/1 -> Add/3
  Shift/1 -> Add2/2
  Add2/1 -> Joint_Output/1
  FS_gain/1 -> Add1/2
  ES_gain/1 -> Add/2
  RG_F_gain/1 -> Sigmoidal MF6/1
  RG_E_gain/1 -> Sigmoidal MF7/1

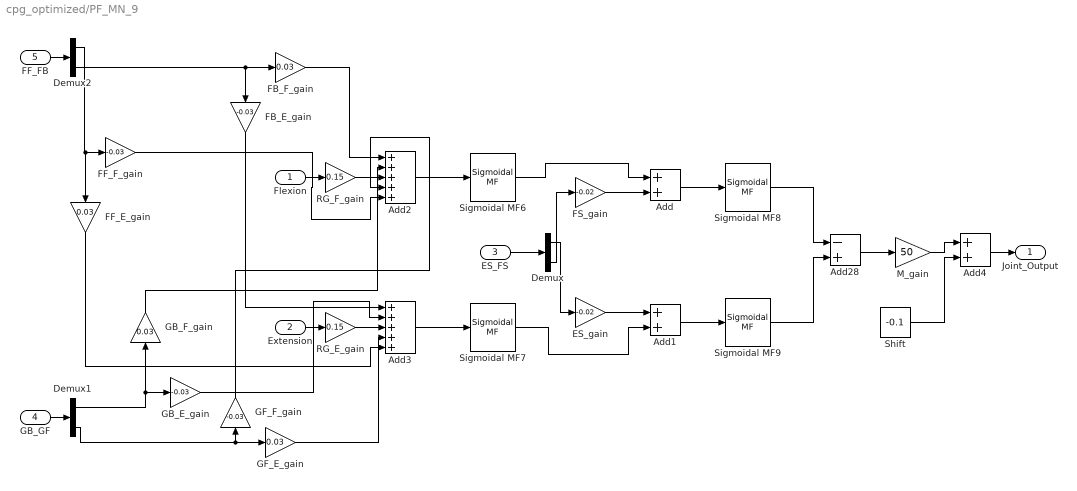
== system cpg_optimized/PF_MN_9 ==
  Flexion : Inport
  Extension : Inport  Port=2
  ES_FS : Inport  Port=3
  GB_GF : Inport  Port=4
  FF_FB : Inport  Port=5
  Add : Sum
  Add1 : Sum
  Add2 : Sum  Inputs=+++++
  Add28 : Sum  Inputs=-+
  Add3 : Sum  Inputs=+++++
  Add4 : Sum
  Demux : Demux  Outputs=2
  Demux1 : Demux  Outputs=2
  Demux2 : Demux  Outputs=2
  ES_gain : Gain  Gain=-0.02
  FB_E_gain : Gain  Gain=-0.03
  FB_F_gain : Gain  Gain=0.03
  FF_E_gain : Gain  Gain=0.03
  FF_F_gain : Gain  Gain=-0.03
  FS_gain : Gain  Gain=-0.02
  GB_E_gain : Gain  Gain=-0.03
  GB_F_gain : Gain  Gain=0.03
  GF_E_gain : Gain  Gain=0.03
  GF_F_gain : Gain  Gain=-0.03
  M_gain : Gain  Gain=50
  RG_E_gain : Gain  Gain=0.15
  RG_F_gain : Gain  Gain=0.15
  Shift : Constant  Value=-0.1
  Sigmoidal MF{6..9} (4 alike) : fuzblock/Membership  Functions/Sigmoidal MF  a=1  c=0
  Joint_Output : Outport
  wires:
  Extension/1 -> RG_E_gain/1
  Flexion/1 -> RG_F_gain/1
  Sigmoidal MF9/1 -> Add28/2
  Sigmoidal MF8/1 -> Add28/1
  Add28/1 -> M_gain/1
  Sigmoidal MF7/1 -> Add1/2
  Add2/1 -> Sigmoidal MF6/1
  Add3/1 -> Sigmoidal MF7/1
  Add1/1 -> Sigmoidal MF9/1
  Add/1 -> Sigmoidal MF8/1
  ES_FS/1 -> Demux/1
  Demux/2 -> FS_gain/1
  Demux/1 -> ES_gain/1
  Sigmoidal MF6/1 -> Add/1
  GB_GF/1 -> Demux1/1
  FF_FB/1 -> Demux2/1
  Demux2/1 -> FF_E_gain/1, FF_F_gain/1
  Demux2/2 -> FB_E_gain/1, FB_F_gain/1
  Demux1/1 -> GB_F_gain/1, GB_E_gain/1
  Demux1/2 -> GF_F_gain/1, GF_E_gain/1
  FS_gain/1 -> Add/2
  ES_gain/1 -> Add1/1
  FB_F_gain/1 -> Add2/1
  FB_E_gain/1 -> Add3/1
  GB_F_gain/1 -> Add2/2
  GB_E_gain/1 -> Add3/2
  GF_E_gain/1 -> Add3/4
  GF_F_gain/1 -> Add2/4
  FF_F_gain/1 -> Add2/5
  FF_E_gain/1 -> Add3/5
  M_gain/1 -> Add4/1
  Shift/1 -> Add4/2
  Add4/1 -> Joint_Output/1
  RG_F_gain/1 -> Add2/3
  RG_E_gain/1 -> Add3/3

== system cpg_optimized/SendJointCommands ==
  Send_Joint_Value? : Inport
  Joint_Value : Inport  Port=2
  Blank Message : robotlib/Blank Message  SourceLibraryInfo=This block requires Robotics System Toolbox  messageType=wrecs_msgs/field_command  SampleTime=inf
  Bus Assignment : BusAssignment  AssignedSignals=SendJointCommand,Position,SetThisJoint
  Constant : Constant  OutDataTypeStr=boolean
  Publish : robotlib/Publish  SourceLibraryInfo=This block requires Robotics System Toolbox  topicSource=Specify your own  topic=/field_command  messageType=wrecs_msgs/field_command  messageQueueLength=1
  wires:
  Blank Message/1 -> Bus Assignment/1
  Bus Assignment/1 -> Publish/1
  Constant/1 -> Bus Assignment/2
  Joint_Value/1 -> Bus Assignment/3
  Send_Joint_Value?/1 -> Bus Assignment/4

== system cpg_optimized/Subsystem4 ==
  MsgIn : Inport
  Enable : EnablePort
  MsgOut : Outport
  wires:
  MsgIn/1 -> MsgOut/1

== system cpg_optimized/cell_10_1 ==
  In1 : Inport
  Add : Sum  Inputs=++-
  Add1 : Sum  Inputs=-+
  Add2 : Sum  Inputs=-+
  DTI_1 : DiscreteIntegrator  InitialCondition=-0.059389  InitialConditionSetting=State (most efficient)  SampleTime=-1  ICPrevOutput=DiscIntNeverNeededParam  ICPrevScaledInput=DiscIntNeverNeededParam
  DTI_2 : DiscreteIntegrator  InitialCondition=-0.031702  InitialConditionSetting=State (most efficient)  SampleTime=-1  ICPrevOutput=DiscIntNeverNeededParam  ICPrevScaledInput=DiscIntNeverNeededParam
  Gain : Gain  Gain=-1/t_m
  Gain1 : Gain  Gain=1/t_s
  Gain2 : Gain  Gain=sigma_s
  Gain3 : Gain  Gain=A_f
  Gain4 : Gain  Gain=sigma_f/A_f
  Trigonometric Function : Trigonometry  Operator=tanh
  Out1 : Outport
  wires:
  Gain/1 -> DTI_1/1
  Add/1 -> Gain/1
  Gain2/1 -> Add1/2
  Gain3/1 -> Add2/1
  Add2/1 -> Add/1
  DTI_1/1 -> Out1/1, Gain2/1, Gain4/1, Add2/2  "V"
  Trigonometric Function/1 -> Gain3/1
  Gain4/1 -> Trigonometric Function/1
  In1/1 -> Add/3
  Add1/1 -> Gain1/1
  Gain1/1 -> DTI_2/1
  DTI_2/1 -> Add1/1, Add/2  "q"

== system cpg_optimized/cell_10_2 ==
  In1 : Inport
  Add : Sum  Inputs=++-
  Add1 : Sum  Inputs=-+
  Add2 : Sum  Inputs=-+
  DTI_1 : DiscreteIntegrator  InitialCondition=0.059389  InitialConditionSetting=State (most efficient)  SampleTime=-1  ICPrevOutput=DiscIntNeverNeededParam  ICPrevScaledInput=DiscIntNeverNeededParam
  DTI_2 : DiscreteIntegrator  InitialCondition=0.031702  InitialConditionSetting=State (most efficient)  SampleTime=-1  ICPrevOutput=DiscIntNeverNeededParam  ICPrevScaledInput=DiscIntNeverNeededParam
  Gain : Gain  Gain=-1/t_m
  Gain1 : Gain  Gain=1/t_s
  Gain2 : Gain  Gain=sigma_s
  Gain3 : Gain  Gain=A_f
  Gain4 : Gain  Gain=sigma_f/A_f
  Trigonometric Function : Trigonometry  Operator=tanh
  Out1 : Outport
  wires:
  Gain/1 -> DTI_1/1
  Add/1 -> Gain/1
  Gain2/1 -> Add1/2
  Gain3/1 -> Add2/1
  Add2/1 -> Add/1
  DTI_1/1 -> Out1/1, Gain2/1, Gain4/1, Add2/2  "V"
  Trigonometric Function/1 -> Gain3/1
  Gain4/1 -> Trigonometric Function/1
  In1/1 -> Add/3
  Add1/1 -> Gain1/1
  Gain1/1 -> DTI_2/1
  DTI_2/1 -> Add1/1, Add/2  "q"

== system cpg_optimized/cell_12_1 ==
  In1 : Inport
  Add : Sum  Inputs=++-
  Add1 : Sum  Inputs=-+
  Add2 : Sum  Inputs=-+
  DTI_1 : DiscreteIntegrator  InitialCondition=0.059357  InitialConditionSetting=State (most efficient)  SampleTime=-1  ICPrevOutput=DiscIntNeverNeededParam  ICPrevScaledInput=DiscIntNeverNeededParam
  DTI_2 : DiscreteIntegrator  InitialCondition=0.031715  InitialConditionSetting=State (most efficient)  SampleTime=-1  ICPrevOutput=DiscIntNeverNeededParam  ICPrevScaledInput=DiscIntNeverNeededParam
  Gain : Gain  Gain=-1/t_m
  Gain1 : Gain  Gain=1/t_s
  Gain2 : Gain  Gain=sigma_s
  Gain3 : Gain  Gain=A_f
  Gain4 : Gain  Gain=sigma_f/A_f
  Trigonometric Function : Trigonometry  Operator=tanh
  Out1 : Outport
  wires:
  Gain/1 -> DTI_1/1
  Add/1 -> Gain/1
  Gain2/1 -> Add1/2
  Gain3/1 -> Add2/1
  Add2/1 -> Add/1
  DTI_1/1 -> Out1/1, Gain2/1, Gain4/1, Add2/2  "V"
  Trigonometric Function/1 -> Gain3/1
  Gain4/1 -> Trigonometric Function/1
  In1/1 -> Add/3
  Add1/1 -> Gain1/1
  Gain1/1 -> DTI_2/1
  DTI_2/1 -> Add1/1, Add/2  "q"

== system cpg_optimized/cell_12_2 ==
  In1 : Inport
  Add : Sum  Inputs=++-
  Add1 : Sum  Inputs=-+
  Add2 : Sum  Inputs=-+
  DTI_1 : DiscreteIntegrator  InitialCondition=-0.059357  InitialConditionSetting=State (most efficient)  SampleTime=-1  ICPrevOutput=DiscIntNeverNeededParam  ICPrevScaledInput=DiscIntNeverNeededParam
  DTI_2 : DiscreteIntegrator  InitialCondition=-0.031715  InitialConditionSetting=State (most efficient)  SampleTime=-1  ICPrevOutput=DiscIntNeverNeededParam  ICPrevScaledInput=DiscIntNeverNeededParam
  Gain : Gain  Gain=-1/t_m
  Gain1 : Gain  Gain=1/t_s
  Gain2 : Gain  Gain=sigma_s
  Gain3 : Gain  Gain=A_f
  Gain4 : Gain  Gain=sigma_f/A_f
  Trigonometric Function : Trigonometry  Operator=tanh
  Out1 : Outport
  wires:
  Gain/1 -> DTI_1/1
  Add/1 -> Gain/1
  Gain2/1 -> Add1/2
  Gain3/1 -> Add2/1
  Add2/1 -> Add/1
  DTI_1/1 -> Out1/1, Gain2/1, Gain4/1, Add2/2  "V"
  Trigonometric Function/1 -> Gain3/1
  Gain4/1 -> Trigonometric Function/1
  In1/1 -> Add/3
  Add1/1 -> Gain1/1
  Gain1/1 -> DTI_2/1
  DTI_2/1 -> Add1/1, Add/2  "q"

== system cpg_optimized/cell_13_1 ==
  In1 : Inport
  Add : Sum  Inputs=++-
  Add1 : Sum  Inputs=-+
  Add2 : Sum  Inputs=-+
  DTI_1 : DiscreteIntegrator  InitialCondition=-0.059359  InitialConditionSetting=State (most efficient)  SampleTime=-1  ICPrevOutput=DiscIntNeverNeededParam  ICPrevScaledInput=DiscIntNeverNeededParam
  DTI_2 : DiscreteIntegrator  InitialCondition=-0.031714  InitialConditionSetting=State (most efficient)  SampleTime=-1  ICPrevOutput=DiscIntNeverNeededParam  ICPrevScaledInput=DiscIntNeverNeededParam
  Gain : Gain  Gain=-1/t_m
  Gain1 : Gain  Gain=1/t_s
  Gain2 : Gain  Gain=sigma_s
  Gain3 : Gain  Gain=A_f
  Gain4 : Gain  Gain=sigma_f/A_f
  Trigonometric Function : Trigonometry  Operator=tanh
  Out1 : Outport
  wires:
  Gain/1 -> DTI_1/1
  Add/1 -> Gain/1
  Gain2/1 -> Add1/2
  Gain3/1 -> Add2/1
  Add2/1 -> Add/1
  DTI_1/1 -> Out1/1, Gain2/1, Gain4/1, Add2/2  "V"
  Trigonometric Function/1 -> Gain3/1
  Gain4/1 -> Trigonometric Function/1
  In1/1 -> Add/3
  Add1/1 -> Gain1/1
  Gain1/1 -> DTI_2/1
  DTI_2/1 -> Add1/1, Add/2  "q"

== system cpg_optimized/cell_13_2 ==
  In1 : Inport
  Add : Sum  Inputs=++-
  Add1 : Sum  Inputs=-+
  Add2 : Sum  Inputs=-+
  DTI_1 : DiscreteIntegrator  InitialCondition=0.059359  InitialConditionSetting=State (most efficient)  SampleTime=-1  ICPrevOutput=DiscIntNeverNeededParam  ICPrevScaledInput=DiscIntNeverNeededParam
  DTI_2 : DiscreteIntegrator  InitialCondition=0.031714  InitialConditionSetting=State (most efficient)  SampleTime=-1  ICPrevOutput=DiscIntNeverNeededParam  ICPrevScaledInput=DiscIntNeverNeededParam
  Gain : Gain  Gain=-1/t_m
  Gain1 : Gain  Gain=1/t_s
  Gain2 : Gain  Gain=sigma_s
  Gain3 : Gain  Gain=A_f
  Gain4 : Gain  Gain=sigma_f/A_f
  Trigonometric Function : Trigonometry  Operator=tanh
  Out1 : Outport
  wires:
  Gain/1 -> DTI_1/1
  Add/1 -> Gain/1
  Gain2/1 -> Add1/2
  Gain3/1 -> Add2/1
  Add2/1 -> Add/1
  DTI_1/1 -> Out1/1, Gain2/1, Gain4/1, Add2/2  "V"
  Trigonometric Function/1 -> Gain3/1
  Gain4/1 -> Trigonometric Function/1
  In1/1 -> Add/3
  Add1/1 -> Gain1/1
  Gain1/1 -> DTI_2/1
  DTI_2/1 -> Add1/1, Add/2  "q"

== system cpg_optimized/cell_14_1 ==
  In1 : Inport
  Add : Sum  Inputs=++-
  Add1 : Sum  Inputs=-+
  Add2 : Sum  Inputs=-+
  DTI_1 : DiscreteIntegrator  InitialCondition=-0.059358  InitialConditionSetting=State (most efficient)  SampleTime=-1  ICPrevOutput=DiscIntNeverNeededParam  ICPrevScaledInput=DiscIntNeverNeededParam
  DTI_2 : DiscreteIntegrator  InitialCondition=-0.031715  InitialConditionSetting=State (most efficient)  SampleTime=-1  ICPrevOutput=DiscIntNeverNeededParam  ICPrevScaledInput=DiscIntNeverNeededParam
  Gain : Gain  Gain=-1/t_m
  Gain1 : Gain  Gain=1/t_s
  Gain2 : Gain  Gain=sigma_s
  Gain3 : Gain  Gain=A_f
  Gain4 : Gain  Gain=sigma_f/A_f
  Trigonometric Function : Trigonometry  Operator=tanh
  Out1 : Outport
  wires:
  Gain/1 -> DTI_1/1
  Add/1 -> Gain/1
  Gain2/1 -> Add1/2
  Gain3/1 -> Add2/1
  Add2/1 -> Add/1
  DTI_1/1 -> Out1/1, Gain2/1, Gain4/1, Add2/2  "V"
  Trigonometric Function/1 -> Gain3/1
  Gain4/1 -> Trigonometric Function/1
  In1/1 -> Add/3
  Add1/1 -> Gain1/1
  Gain1/1 -> DTI_2/1
  DTI_2/1 -> Add1/1, Add/2  "q"

== system cpg_optimized/cell_14_2 ==
  In1 : Inport
  Add : Sum  Inputs=++-
  Add1 : Sum  Inputs=-+
  Add2 : Sum  Inputs=-+
  DTI_1 : DiscreteIntegrator  InitialCondition=0.059358  InitialConditionSetting=State (most efficient)  SampleTime=-1  ICPrevOutput=DiscIntNeverNeededParam  ICPrevScaledInput=DiscIntNeverNeededParam
  DTI_2 : DiscreteIntegrator  InitialCondition=0.031715  InitialConditionSetting=State (most efficient)  SampleTime=-1  ICPrevOutput=DiscIntNeverNeededParam  ICPrevScaledInput=DiscIntNeverNeededParam
  Gain : Gain  Gain=-1/t_m
  Gain1 : Gain  Gain=1/t_s
  Gain2 : Gain  Gain=sigma_s
  Gain3 : Gain  Gain=A_f
  Gain4 : Gain  Gain=sigma_f/A_f
  Trigonometric Function : Trigonometry  Operator=tanh
  Out1 : Outport
  wires:
  Gain/1 -> DTI_1/1
  Add/1 -> Gain/1
  Gain2/1 -> Add1/2
  Gain3/1 -> Add2/1
  Add2/1 -> Add/1
  DTI_1/1 -> Out1/1, Gain2/1, Gain4/1, Add2/2  "V"
  Trigonometric Function/1 -> Gain3/1
  Gain4/1 -> Trigonometric Function/1
  In1/1 -> Add/3
  Add1/1 -> Gain1/1
  Gain1/1 -> DTI_2/1
  DTI_2/1 -> Add1/1, Add/2  "q"

== system cpg_optimized/cell_15_1 ==
  In1 : Inport
  Add : Sum  Inputs=++-
  Add1 : Sum  Inputs=-+
  Add2 : Sum  Inputs=-+
  DTI_1 : DiscreteIntegrator  InitialCondition=0.059349  InitialConditionSetting=State (most efficient)  SampleTime=-1  ICPrevOutput=DiscIntNeverNeededParam  ICPrevScaledInput=DiscIntNeverNeededParam
  DTI_2 : DiscreteIntegrator  InitialCondition=0.031718  InitialConditionSetting=State (most efficient)  SampleTime=-1  ICPrevOutput=DiscIntNeverNeededParam  ICPrevScaledInput=DiscIntNeverNeededParam
  Gain : Gain  Gain=-1/t_m
  Gain1 : Gain  Gain=1/t_s
  Gain2 : Gain  Gain=sigma_s
  Gain3 : Gain  Gain=A_f
  Gain4 : Gain  Gain=sigma_f/A_f
  Trigonometric Function : Trigonometry  Operator=tanh
  Out1 : Outport
  wires:
  Gain/1 -> DTI_1/1
  Add/1 -> Gain/1
  Gain2/1 -> Add1/2
  Gain3/1 -> Add2/1
  Add2/1 -> Add/1
  DTI_1/1 -> Out1/1, Gain2/1, Gain4/1, Add2/2  "V"
  Trigonometric Function/1 -> Gain3/1
  Gain4/1 -> Trigonometric Function/1
  In1/1 -> Add/3
  Add1/1 -> Gain1/1
  Gain1/1 -> DTI_2/1
  DTI_2/1 -> Add1/1, Add/2  "q"

== system cpg_optimized/cell_15_2 ==
  In1 : Inport
  Add : Sum  Inputs=++-
  Add1 : Sum  Inputs=-+
  Add2 : Sum  Inputs=-+
  DTI_1 : DiscreteIntegrator  InitialCondition=-0.059349  InitialConditionSetting=State (most efficient)  SampleTime=-1  ICPrevOutput=DiscIntNeverNeededParam  ICPrevScaledInput=DiscIntNeverNeededParam
  DTI_2 : DiscreteIntegrator  InitialCondition=-0.031718  InitialConditionSetting=State (most efficient)  SampleTime=-1  ICPrevOutput=DiscIntNeverNeededParam  ICPrevScaledInput=DiscIntNeverNeededParam
  Gain : Gain  Gain=-1/t_m
  Gain1 : Gain  Gain=1/t_s
  Gain2 : Gain  Gain=sigma_s
  Gain3 : Gain  Gain=A_f
  Gain4 : Gain  Gain=sigma_f/A_f
  Trigonometric Function : Trigonometry  Operator=tanh
  Out1 : Outport
  wires:
  Gain/1 -> DTI_1/1
  Add/1 -> Gain/1
  Gain2/1 -> Add1/2
  Gain3/1 -> Add2/1
  Add2/1 -> Add/1
  DTI_1/1 -> Out1/1, Gain2/1, Gain4/1, Add2/2  "V"
  Trigonometric Function/1 -> Gain3/1
  Gain4/1 -> Trigonometric Function/1
  In1/1 -> Add/3
  Add1/1 -> Gain1/1
  Gain1/1 -> DTI_2/1
  DTI_2/1 -> Add1/1, Add/2  "q"

== system cpg_optimized/cell_16_1 ==
  In1 : Inport
  Add : Sum  Inputs=++-
  Add1 : Sum  Inputs=-+
  Add2 : Sum  Inputs=-+
  DTI_1 : DiscreteIntegrator  InitialCondition=0.05931  InitialConditionSetting=State (most efficient)  SampleTime=-1  ICPrevOutput=DiscIntNeverNeededParam  ICPrevScaledInput=DiscIntNeverNeededParam
  DTI_2 : DiscreteIntegrator  InitialCondition=0.031734  InitialConditionSetting=State (most efficient)  SampleTime=-1  ICPrevOutput=DiscIntNeverNeededParam  ICPrevScaledInput=DiscIntNeverNeededParam
  Gain : Gain  Gain=-1/t_m
  Gain1 : Gain  Gain=1/t_s
  Gain2 : Gain  Gain=sigma_s
  Gain3 : Gain  Gain=A_f
  Gain4 : Gain  Gain=sigma_f/A_f
  Trigonometric Function : Trigonometry  Operator=tanh
  Out1 : Outport
  wires:
  Gain/1 -> DTI_1/1
  Add/1 -> Gain/1
  Gain2/1 -> Add1/2
  Gain3/1 -> Add2/1
  Add2/1 -> Add/1
  DTI_1/1 -> Out1/1, Gain2/1, Gain4/1, Add2/2  "V"
  Trigonometric Function/1 -> Gain3/1
  Gain4/1 -> Trigonometric Function/1
  In1/1 -> Add/3
  Add1/1 -> Gain1/1
  Gain1/1 -> DTI_2/1
  DTI_2/1 -> Add1/1, Add/2  "q"

== system cpg_optimized/cell_16_2 ==
  In1 : Inport
  Add : Sum  Inputs=++-
  Add1 : Sum  Inputs=-+
  Add2 : Sum  Inputs=-+
  DTI_1 : DiscreteIntegrator  InitialCondition=-0.05931  InitialConditionSetting=State (most efficient)  SampleTime=-1  ICPrevOutput=DiscIntNeverNeededParam  ICPrevScaledInput=DiscIntNeverNeededParam
  DTI_2 : DiscreteIntegrator  InitialCondition=-0.031734  InitialConditionSetting=State (most efficient)  SampleTime=-1  ICPrevOutput=DiscIntNeverNeededParam  ICPrevScaledInput=DiscIntNeverNeededParam
  Gain : Gain  Gain=-1/t_m
  Gain1 : Gain  Gain=1/t_s
  Gain2 : Gain  Gain=sigma_s
  Gain3 : Gain  Gain=A_f
  Gain4 : Gain  Gain=sigma_f/A_f
  Trigonometric Function : Trigonometry  Operator=tanh
  Out1 : Outport
  wires:
  Gain/1 -> DTI_1/1
  Add/1 -> Gain/1
  Gain2/1 -> Add1/2
  Gain3/1 -> Add2/1
  Add2/1 -> Add/1
  DTI_1/1 -> Out1/1, Gain2/1, Gain4/1, Add2/2  "V"
  Trigonometric Function/1 -> Gain3/1
  Gain4/1 -> Trigonometric Function/1
  In1/1 -> Add/3
  Add1/1 -> Gain1/1
  Gain1/1 -> DTI_2/1
  DTI_2/1 -> Add1/1, Add/2  "q"

== system cpg_optimized/cell_18_1 ==
  In1 : Inport
  Add : Sum  Inputs=++-
  Add1 : Sum  Inputs=-+
  Add2 : Sum  Inputs=-+
  DTI_1 : DiscreteIntegrator  InitialCondition=-0.065208  InitialConditionSetting=State (most efficient)  SampleTime=-1  ICPrevOutput=DiscIntNeverNeededParam  ICPrevScaledInput=DiscIntNeverNeededParam
  DTI_2 : DiscreteIntegrator  InitialCondition=-0.029689  InitialConditionSetting=State (most efficient)  SampleTime=-1  ICPrevOutput=DiscIntNeverNeededParam  ICPrevScaledInput=DiscIntNeverNeededParam
  Gain : Gain  Gain=-1/t_m
  Gain1 : Gain  Gain=1/t_s
  Gain2 : Gain  Gain=sigma_s
  Gain3 : Gain  Gain=A_f
  Gain4 : Gain  Gain=sigma_f/A_f
  Trigonometric Function : Trigonometry  Operator=tanh
  Out1 : Outport
  wires:
  Gain/1 -> DTI_1/1
  Add/1 -> Gain/1
  Gain2/1 -> Add1/2
  Gain3/1 -> Add2/1
  Add2/1 -> Add/1
  DTI_1/1 -> Out1/1, Gain2/1, Gain4/1, Add2/2  "V"
  Trigonometric Function/1 -> Gain3/1
  Gain4/1 -> Trigonometric Function/1
  In1/1 -> Add/3
  Add1/1 -> Gain1/1
  Gain1/1 -> DTI_2/1
  DTI_2/1 -> Add1/1, Add/2  "q"
